simulink model "IndustrialMicrogrid"  (R2025a)
settings: Solver=FixedStepAuto  StartTime=0.0  StopTime=8  FixedStep=Ts  RelTol=1e-3
PostLoadFcn:
  | IndustrialMicrogridInputData
  | GfmGridFormingConverterInputParameters
model workspace (MAT data in the model file):
  caseNum = 2
undefined symbols (not defined in the file): base, BESS, DiscIntNeverNeededParam, grid, Grid, gridInverter, machine, microgrid, PV, PVInverter, PVTransformer, scrFactorRg, scrFactorXg, transformer, Transition_and_Dispatch_ControlModeType, Ts
libraries: ee_lib x126, fl_lib x91, eeGeneralControl x73, nesl_utility x50, nesl_utility_internal x46, simulink x30, eeTransforms x11, eeSinusoidalMeasurementV2 x5, eeTotalHarmonicDistorsion x4, slpidlib x3, simulink_extras x2, eePowerMeasurement x2
(part 3 of 12)

== system IndustrialMicrogrid/MG1 Drilling Loads/Subsystem2 ==
  ASM measurement : ee_lib/Electromechanical/Asynchronous/Induction Machine Measurement  output_idx=11
      settings: InternalSimscapePortConfiguration="{\"Bottom\":[],\"Left\":[{\"id\":\"pu_input\",\"label\":\"pu\",\"type\":\"input\"}],\"Right\":[{\"id\":\"pu_output\",\"label\":\"o\",\"type\":\"output\"}],\"Top\":[]}"
  ASM measurement1 : ee_lib/Electromechanical/Asynchronous/Induction Machine Measurement  output_idx=12
      settings: InternalSimscapePortConfiguration="{\"Bottom\":[],\"Left\":[{\"id\":\"pu_input\",\"label\":\"pu\",\"type\":\"input\"}],\"Right\":[{\"id\":\"pu_output\",\"label\":\"o\",\"type\":\"output\"}],\"Top\":[]}"
  ASM measurement2 : ee_lib/Electromechanical/Asynchronous/Induction Machine Measurement  output_idx=12
      settings: InternalSimscapePortConfiguration="{\"Bottom\":[],\"Left\":[{\"id\":\"pu_input\",\"label\":\"pu\",\"type\":\"input\"}],\"Right\":[{\"id\":\"pu_output\",\"label\":\"o\",\"type\":\"output\"}],\"Top\":[]}"
  Asynchronous Machine Squirrel Cage (fundamental) : ee_lib/Electromechanical/Asynchronous/Induction Machine Squirrel Cage  port_option=ee.enum.threePhasePort.composite  SRated=132000 V*A  VRated=microgrid.unitSubstationVoltage V  FRated=grid.frequency Hz  nPolePairs=2  param_unit=ee.enum.unit.si  squirrel_cage=ee.enum.squirrelcage.Single  zero_sequence=ee.enum.park.zerosequence.exclude  initialization_option=ee.enum.asm.initialization.fluxvariables  Rs=0.016744 Ohm  Xls=0.035490 Ohm  pu_Rs=0.0258  pu_Lls=0.0413  Rrd=0.009857 Ohm  Xlrd=0.04280 Ohm  pu_Rrd=0.0145  pu_Llrd=0.0424  Rrd1=0.28 Ohm  Xlrd1=0.82 Ohm  Rrd2=0.28 Ohm  Xlrd2=0.82 Ohm  pu_Rrd1=0.0290  pu_Llrd1=0.0848  pu_Rrd2=0.0290  pu_Llrd2=0.0848  Xm=111.90 Ohm  pu_Lm=1.7562  X0=0.4 Ohm  pu_L0=0.0413  saturation_option=ee.enum.saturation.exclude  saturation_i=[0, 4, 9, 18, 25, 34, 50, 68, 95, 120] A  saturation_v=[0, 88, 154, 198, 220, 242, 264, 286, 308, 327] V  pu_saturation_i=[0, .176, .396, .792, 1.1, 1.496, 2.2, 2.992, 4.18, 5.28]  pu_saturation_v=[0, .4, .7, .9, 1, 1.1, 1.2, 1.3, 1.4, 1.4864]  connection_option=ee.enum.Connection.delta1  angular_position_specify=off  angular_position_priority=None  angular_position=0 deg  angular_position_nominal_specify=off  angular_position_nominal_value=1  angular_position_nominal_unit=deg  pu_psids_specify=off  pu_psids_priority=None  pu_psids=0  pu_psids_nominal_specify=off  pu_psids_nominal_value=1  pu_psids_nominal_unit=1  pu_psiqs_specify=off  pu_psiqs_priority=None  pu_psiqs=0  pu_psiqs_nominal_specify=off  pu_psiqs_nominal_value=1  pu_psiqs_nominal_unit=1  pu_psi0s_specify=off  pu_psi0s_priority=None  pu_psi0s=0  pu_psi0s_nominal_specify=off  pu_psi0s_nominal_value=1  pu_psi0s_nominal_unit=1  pu_psidr_specify=off  pu_psidr_priority=None  pu_psidr=0  pu_psidr_nominal_specify=off  pu_psidr_nominal_value=1  pu_psidr_nominal_unit=1  pu_psiqr_specify=off  pu_psiqr_priority=None  pu_psiqr=0  pu_psiqr_nominal_specify=off  pu_psiqr_nominal_value=1  pu_psiqr_nominal_unit=1  pu_psidr1_specify=off  pu_psidr1_priority=None  pu_psidr1=0  pu_psidr1_nominal_specify=off  pu_psidr1_nominal_value=1  pu_psidr1_nominal_unit=1  pu_psiqr1_specify=off  pu_psiqr1_priority=None  pu_psiqr1=0  pu_psiqr1_nominal_specify=off  pu_psiqr1_nominal_value=1  pu_psiqr1_nominal_unit=1  pu_psidr2_specify=off  pu_psidr2_priority=None  pu_psidr2=0  pu_psidr2_nominal_specify=off  pu_psidr2_nominal_value=1  pu_psidr2_nominal_unit=1  pu_psiqr2_specify=off  pu_psiqr2_priority=None  pu_psiqr2=0  pu_psiqr2_nominal_specify=off  pu_psiqr2_nominal_value=1  pu_psiqr2_nominal_unit=1  psids_specify=off  psids_priority=None  psids=0 Wb  psids_nominal_specify=off  psids_nominal_value=1  psids_nominal_unit=Wb  psiqs_specify=off  psiqs_priority=None  psiqs=0 Wb  psiqs_nominal_specify=off  psiqs_nominal_value=1  psiqs_nominal_unit=Wb  psi0s_specify=off  psi0s_priority=None  psi0s=0 Wb  psi0s_nominal_specify=off  psi0s_nominal_value=1  psi0s_nominal_unit=Wb  psidr_specify=off  psidr_priority=None  psidr=0 Wb  psidr_nominal_specify=off  psidr_nominal_value=1  psidr_nominal_unit=Wb  psiqr_specify=off  psiqr_priority=None  psiqr=0 Wb  psiqr_nominal_specify=off  psiqr_nominal_value=1  psiqr_nominal_unit=Wb  psidr1_specify=off  psidr1_priority=None  psidr1=0 Wb  psidr1_nominal_specify=off  psidr1_nominal_value=1  psidr1_nominal_unit=Wb  psiqr1_specify=off  psiqr1_priority=None  psiqr1=0 Wb  psiqr1_nominal_specify=off  psiqr1_nominal_value=1  psiqr1_nominal_unit=Wb  psidr2_specify=off  psidr2_priority=None  psidr2=0 Wb  psidr2_nominal_specify=off  psidr2_nominal_value=1  psidr2_nominal_unit=Wb  psiqr2_specify=off  psiqr2_priority=None  psiqr2=0 Wb  psiqr2_nominal_specify=off  psiqr2_nominal_value=1  psiqr2_nominal_unit=Wb  slip_specify=off  slip_priority=None  slip=0  slip_nominal_specify=off  slip_nominal_value=1  slip_nominal_unit=1  real_power_generated_specify=off  real_power_generated_priority=None  real_power_generated=0 W  real_power_generated_nominal_specify=off  real_power_generated_nominal_value=1  real_power_generated_nominal_unit=W  mechanical_power_consumed_specify=off  mechanical_power_consumed_priority=None  mechanical_power_consumed=0 W  mechanical_power_consumed_nominal_specify=off  mechanical_power_consumed_nominal_value=1  mechanical_power_consumed_nominal_unit=W  Tmeas=298.15 K  alpha=3.93e-3 1/K  alpha_cage=4.4e-3 1/K  stator_thermal_mass=100 J/K  rotor_thermal_mass=200 J/K  temperatureA_specify=off  temperatureA_priority=High  temperatureA=25 degC  temperatureA_nominal_specify=off  temperatureA_nominal_value=1  temperatureA_nominal_unit=degC  temperatureB_specify=off  temperatureB_priority=High  temperatureB=25 degC  temperatureB_nominal_specify=off  temperatureB_nominal_value=1  temperatureB_nominal_unit=degC  temperatureC_specify=off  temperatureC_priority=High  temperatureC=25 degC  temperatureC_nominal_specify=off  temperatureC_nominal_value=1  temperatureC_nominal_unit=degC  temperatureR_specify=off  temperatureR_priority=High  temperatureR=25 degC  temperatureR_nominal_specify=off  temperatureR_nominal_value=1  temperatureR_nominal_unit=degC
      settings: InternalSimscapePortConfiguration="{\"Bottom\":[],\"Left\":[{\"id\":\"R\",\"label\":\"R\",\"type\":\"foundation.mechanical.rotational.rotational\"},{\"id\":\"C\",\"label\":\"C\",\"type\":\"foundation.mechanical.rotational.rotational\"}],\"Right\":[{\"id\":\"pu_output\",\"label\":\"pu\",\"type\":\"output\"},{\"id\":\"N1\",\"label\":\"~1\",\"type\":\"foundation.electrical.three_phase\"},{\"id\":\"N2\",\"label\":\"~2\",\"type\":\"foundation.electrical.three_phase\"}],\"Top\":[]}"
  Electrical Reference1 : fl_lib/Electrical/Electrical Elements/Electrical Reference
  Generator : Scope  NumInputPorts=3
      settings: TimeSpan=60  ActiveDisplayYMinimum=-4.80755  ActiveDisplayYMaximum=1.91952  DataLoggingVariableName=ScopeData2  DataLoggingSaveFormat=Array
  Generator Sign Convention : Gain  Gain=-1
  Generator Sign Convention1 : Gain  Gain=-1
  Neutral Port (Three-Phase) : ee_lib/Connectors & References/Neutral Port (Three-Phase)  G_parasitic=1e-12 1/Ohm
      settings: InternalSimscapePortConfiguration="{\"Bottom\":[],\"Left\":[{\"id\":\"N\",\"label\":\"~\",\"type\":\"foundation.electrical.three_phase\"}],\"Right\":[{\"id\":\"n\",\"label\":\"n\",\"type\":\"foundation.electrical.electrical\"}],\"Top\":[]}"
  PS-Simulink Converter1 : nesl_utility/PS-Simulink Converter  PhysicalDomain=network_engine_domain  SubClassName=ps_output  LeftPortType=input  RightPortType=output  PseudoPeriodic=off  Frequencies=[]  VectorFormat=1-D array  Unit=1  AffineConversion=off
  PS-Simulink Converter2 : nesl_utility/PS-Simulink Converter  PhysicalDomain=network_engine_domain  SubClassName=ps_output  LeftPortType=input  RightPortType=output  PseudoPeriodic=off  Frequencies=[]  VectorFormat=1-D array  Unit=1  AffineConversion=off
  PS-Simulink Converter3 : nesl_utility/PS-Simulink Converter  PhysicalDomain=network_engine_domain  SubClassName=ps_output  LeftPortType=input  RightPortType=output  PseudoPeriodic=off  Frequencies=[]  VectorFormat=1-D array  Unit=1  AffineConversion=off
  Subsystem : Subsystem
  Conn2 : PMIOPort  Side=Right
  wires:
  PS-Simulink Converter3/1 -> Generator/3
  Generator Sign Convention1/1 -> Generator/2  "Reactive Power, pu"
  PS-Simulink Converter2/1 -> Generator Sign Convention/1
  Generator Sign Convention/1 -> Generator/1  "Real Power, pu"
  PS-Simulink Converter1/1 -> Generator Sign Convention1/1
  connections:
  ASM measurement1/RConn1 -- PS-Simulink Converter1/LConn1
  PS-Simulink Converter3/LConn1 -- ASM measurement2/RConn1
  Asynchronous Machine Squirrel Cage (fundamental)/RConn3 -- Neutral Port (Three-Phase)/LConn1
  Asynchronous Machine Squirrel Cage (fundamental)/RConn2 -- Conn2/RConn1
  ASM measurement/RConn1 -- PS-Simulink Converter2/LConn1
  Neutral Port (Three-Phase)/RConn1 -- Electrical Reference1/LConn1
  Subsystem/LConn1 -- Asynchronous Machine Squirrel Cage (fundamental)/LConn1
  Subsystem/LConn2 -- Asynchronous Machine Squirrel Cage (fundamental)/LConn2
  ASM measurement1/LConn1 -- ASM measurement2/LConn1 -- Asynchronous Machine Squirrel Cage (fundamental)/RConn1 -- ASM measurement/LConn1

== system IndustrialMicrogrid/MG1 Portable Substation/Circuit Breaker1 ==
  BRK : Inport
  Data Type Conversion : DataTypeConversion  OutDataTypeStr=double  SaturateOnIntegerOverflow=off  RndMeth=Floor
  Open Resistance : Gain  Gain=1e5
  Phase Splitter : ee_lib/Connectors & References/Phase Splitter
  Phase Splitter1 : ee_lib/Connectors & References/Phase Splitter
  Simulink-PS Converter : nesl_utility/Simulink-PS Converter  PhysicalDomain=network_engine_domain  SubClassName=ps_input  LeftPortType=input  RightPortType=output  PseudoPeriodic=off  Frequencies=[]  NoiseDistribution=none  NoiseParameters=[]  Unit=1  AffineConversion=off  FilteringAndDerivatives=provide  SimscapeFilterOrder=1  InputFilterTimeConstant=0.001  UdotUserProvided=0
  Variable Resistor : fl_lib/Electrical/Electrical Elements/Variable Resistor  Rmin=1e-3 Ohm  thermalEnable=false  thermal_mass=1 J/K  i_specify=off  i_priority=None  i=0 A  i_nominal_specify=off  i_nominal_value=1  i_nominal_unit=A  v_specify=off  v_priority=None  v=0 V  v_nominal_specify=off  v_nominal_value=1  v_nominal_unit=V  T_specify=off  T_priority=None  T=300 K  T_nominal_specify=off  T_nominal_value=1  T_nominal_unit=K
  Variable Resistor1 : fl_lib/Electrical/Electrical Elements/Variable Resistor  Rmin=1e-3 Ohm  thermalEnable=false  thermal_mass=1 J/K  i_specify=off  i_priority=None  i=0 A  i_nominal_specify=off  i_nominal_value=1  i_nominal_unit=A  v_specify=off  v_priority=None  v=0 V  v_nominal_specify=off  v_nominal_value=1  v_nominal_unit=V  T_specify=off  T_priority=None  T=300 K  T_nominal_specify=off  T_nominal_value=1  T_nominal_unit=K
  Variable Resistor2 : fl_lib/Electrical/Electrical Elements/Variable Resistor  Rmin=1e-3 Ohm  thermalEnable=false  thermal_mass=1 J/K  i_specify=off  i_priority=None  i=0 A  i_nominal_specify=off  i_nominal_value=1  i_nominal_unit=A  v_specify=off  v_priority=None  v=0 V  v_nominal_specify=off  v_nominal_value=1  v_nominal_unit=V  T_specify=off  T_priority=None  T=300 K  T_nominal_specify=off  T_nominal_value=1  T_nominal_unit=K
  In : PMIOPort  Side=Left
  ~ : PMIOPort  Port=2  Side=Right
  wires:
  Data Type Conversion/1 -> Open Resistance/1
  BRK/1 -> Data Type Conversion/1
  Open Resistance/1 -> Simulink-PS Converter/1
  connections:
  Phase Splitter1/RConn2 -- Variable Resistor1/RConn1
  Variable Resistor1/LConn2 -- Phase Splitter/RConn2
  Phase Splitter1/RConn3 -- Variable Resistor2/RConn1
  Phase Splitter/RConn1 -- Variable Resistor/LConn2
  Variable Resistor2/LConn2 -- Phase Splitter/RConn3
  Phase Splitter1/RConn1 -- Variable Resistor/RConn1
  Phase Splitter1/LConn1 -- ~/RConn1
  Variable Resistor/LConn1 -- Simulink-PS Converter/RConn1 -- Variable Resistor2/LConn1 -- Variable Resistor1/LConn1
  Phase Splitter/LConn1 -- In/RConn1

== system IndustrialMicrogrid/MG1 Primary Substation/BESS and Controller ==
  CntrlRmIN : Inport
  Vref : Inport  Port=2
  f0 : Inport  Port=3
  PQref : Inport  Port=4
  BESS : Subsystem
      settings: PortSchema="{\"entries\":[{\"content\":{\"sides\":[{\"content\":{\"connectorIds\":[\"LConn1\"]},\"type\":\"ConnectorPlacement.EquallySpacedRectSide\",\"uuid\":\"2696dcad-9c9f-4771-9a46-e4805fbfd4e9\"},{\"content\":{\"connectorIds\":[\"In1\",\"In2\",\"In3\",\"In4\"],\"side\":\"RIGHT\"},\"type\":\"ConnectorPlacement.EquallySpacedRectSide\",\"uuid\":\"645d6df5-6573-4261-af42-019db177e35c\"},{\"content\":{\"side\":\"TOP\"},\"type\":\"ConnectorPlacement.EquallySpacedRectSide\",\"uuid\":\"6dbeb1fb-6f20-4035-89b5-3497a08373ed\"}]},\"type\":\"ConnectorPlacement.EquallySpacedConnector\",\"uuid\":\"8e6ce7c3-5a23-40aa-ad05-ea5cef07dce4\"}],\"packageUris\":[\"http://schema.mathworks.com/mf0/Connector/R2020b\"],\"version\":\"1.0\"}"
  "BESS Converter Measurement " : Subsystem
  BESS output filter and transformer1 : Subsystem
  Gain : Gain  Gain=1/grid.frequency
  ~ : PMIOPort  Side=Left
  mBESS : Outport
  wires:
  PQref/1 -> BESS/2(PQref)
  "BESS Converter Measurement "/1(mBESS1) -> mBESS/1
  Vref/1 -> BESS/3(Vref)
  f0/1 -> Gain/1
  CntrlRmIN/1 -> BESS/1(CntrlRmIN1)
  Gain/1 -> BESS/4(f0)
  connections:
  BESS output filter and transformer1/RConn1 -- "BESS Converter Measurement "/LConn1
  BESS/LConn1 -- BESS output filter and transformer1/LConn1
  ~/RConn1 -- "BESS Converter Measurement "/RConn1

== system IndustrialMicrogrid/MG1 Primary Substation/Circuit Breaker1 ==
  BRK : Inport
  Data Type Conversion : DataTypeConversion  OutDataTypeStr=double  SaturateOnIntegerOverflow=off  RndMeth=Floor
  Open Resistance : Gain  Gain=1e5
  Phase Splitter : ee_lib/Connectors & References/Phase Splitter
  Phase Splitter1 : ee_lib/Connectors & References/Phase Splitter
  Simulink-PS Converter : nesl_utility/Simulink-PS Converter  PhysicalDomain=network_engine_domain  SubClassName=ps_input  LeftPortType=input  RightPortType=output  PseudoPeriodic=off  Frequencies=[]  NoiseDistribution=none  NoiseParameters=[]  Unit=1  AffineConversion=off  FilteringAndDerivatives=provide  SimscapeFilterOrder=1  InputFilterTimeConstant=0.001  UdotUserProvided=0
  Variable Resistor : fl_lib/Electrical/Electrical Elements/Variable Resistor  Rmin=1e-3 Ohm  thermalEnable=false  thermal_mass=1 J/K  i_specify=off  i_priority=None  i=0 A  i_nominal_specify=off  i_nominal_value=1  i_nominal_unit=A  v_specify=off  v_priority=None  v=0 V  v_nominal_specify=off  v_nominal_value=1  v_nominal_unit=V  T_specify=off  T_priority=None  T=300 K  T_nominal_specify=off  T_nominal_value=1  T_nominal_unit=K
  Variable Resistor1 : fl_lib/Electrical/Electrical Elements/Variable Resistor  Rmin=1e-3 Ohm  thermalEnable=false  thermal_mass=1 J/K  i_specify=off  i_priority=None  i=0 A  i_nominal_specify=off  i_nominal_value=1  i_nominal_unit=A  v_specify=off  v_priority=None  v=0 V  v_nominal_specify=off  v_nominal_value=1  v_nominal_unit=V  T_specify=off  T_priority=None  T=300 K  T_nominal_specify=off  T_nominal_value=1  T_nominal_unit=K
  Variable Resistor2 : fl_lib/Electrical/Electrical Elements/Variable Resistor  Rmin=1e-3 Ohm  thermalEnable=false  thermal_mass=1 J/K  i_specify=off  i_priority=None  i=0 A  i_nominal_specify=off  i_nominal_value=1  i_nominal_unit=A  v_specify=off  v_priority=None  v=0 V  v_nominal_specify=off  v_nominal_value=1  v_nominal_unit=V  T_specify=off  T_priority=None  T=300 K  T_nominal_specify=off  T_nominal_value=1  T_nominal_unit=K
  In : PMIOPort  Side=Left
  ~ : PMIOPort  Port=2  Side=Right
  wires:
  Data Type Conversion/1 -> Open Resistance/1
  Open Resistance/1 -> Simulink-PS Converter/1
  BRK/1 -> Data Type Conversion/1
  connections:
  Phase Splitter1/RConn2 -- Variable Resistor1/RConn1
  Variable Resistor1/LConn2 -- Phase Splitter/RConn2
  Phase Splitter1/RConn3 -- Variable Resistor2/RConn1
  Phase Splitter/RConn1 -- Variable Resistor/LConn2
  Variable Resistor2/LConn2 -- Phase Splitter/RConn3
  Phase Splitter1/RConn1 -- Variable Resistor/RConn1
  Phase Splitter1/LConn1 -- ~/RConn1
  Variable Resistor/LConn1 -- Simulink-PS Converter/RConn1 -- Variable Resistor2/LConn1 -- Variable Resistor1/LConn1
  Phase Splitter/LConn1 -- In/RConn1

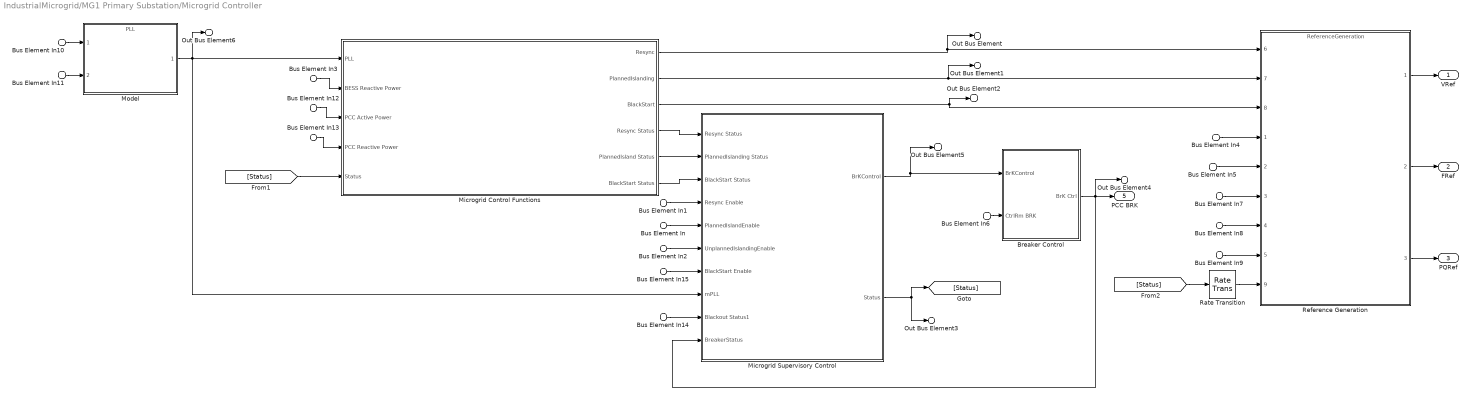
== system IndustrialMicrogrid/MG1 Primary Substation/Microgrid Controller ==
  Bus Element In3 : Inport  PortName=CtrlRm  Element=BESSReactivePower
  Bus Element In9 : Inport  PortName=CtrlRm  Element=PowerCmd
  Bus Element In : Inport  PortName=CtrlRm  Element=plannedIslanding
  Bus Element In2 : Inport  PortName=CtrlRm  Element=unplannedIslanding
  Bus Element In6 : Inport  PortName=CtrlRm  Element=BRKcontrol
  Bus Element In1 : Inport  PortName=CtrlRm  Element=Resync
  Bus Element In4 : Inport  PortName=CtrlRm  Element=BESS.PRef
  Bus Element In5 : Inport  PortName=CtrlRm  Element=BESS.QRef
  Bus Element In7 : Inport  PortName=CtrlRm  Element=BESS.VRef
  Bus Element In8 : Inport  PortName=CtrlRm  Element=BESS.FRef
  Bus Element In15 : Inport  PortName=CtrlRm  Element=blackStart
  Bus Element In14 : Inport  PortName=CtrlRm  Element=blackout
  Bus Element In10 : Inport  Port=2  PortName=mPCC  Element=Grid.voltage
  Bus Element In11 : Inport  Port=2  PortName=mPCC  Element=PCC.voltage
  Bus Element In12 : Inport  Port=2  PortName=mPCC  Element=PCC.activePower
  Bus Element In13 : Inport  Port=2  PortName=mPCC  Element=PCC.reactivePower
  Breaker Control : Subsystem  mask(Breaker Control){}
      mask help: Control breaker at PCC
  Microgrid Control Functions : Subsystem
  Microgrid Supervisory Control : Subsystem
  Model : ModelReference  ModelNameDialog=PLL.slx  UsingDefaultArgumentValue=0,0,0  SimulationMode=Normal  ModelReferenceVersion=5.0  GridFrequency=gridFrequency  KiPLLController=kpPLL  KpPLLController=kiPLL
  Rate Transition : RateTransition  OutPortSampleTime=1e-3
  Reference Generation : ModelReference  ModelNameDialog=ReferenceGeneration.slx  UsingDefaultArgumentValue=0,0,0,0,0  SimulationMode=Normal  ModelReferenceVersion=5.0  GridFrequency=gridFrequency  pUpperLimit=pUpperLimit  pLowerLimit=pLowerLimit  qUpperLimit=qUpperLimit  qLowerLimit=qLowerLimit
      settings: PortSchema="{\"entries\":[{\"content\":{\"sides\":[{\"content\":{\"connectorIds\":[\"In6\",\"In7\",\"In8\",\"In1\",\"In2\",\"In3\",\"In4\",\"In5\",\"In9\"]},\"type\":\"ConnectorPlacement.EquallySpacedRectSide\",\"uuid\":\"e872b833-49f6-4912-b4b3-51343786db27\"},{\"content\":{\"connectorIds\":[\"Out1\",\"Out2\",\"Out3\"],\"side\":\"RIGHT\"},\"type\":\"ConnectorPlacement.EquallySpacedRectSide\",\"uuid\":\"d01ecec0-b655-4b5d-a34d-324f522879ad\"},{\"content\":{\"side\":\"TOP\"},\"type\":\"ConnectorPlacement.EquallySpacedRectSide\",\"uuid\":\"07b88f4e-1122-4691-94e1-fc20c2cbb47d\"}]},\"type\":\"ConnectorPlacement.EquallySpacedConnector\",\"uuid\":\"8d1da379-bdae-48c1-83d9-0dc3b93882b1\"}],\"packageUris\":[\"http://schema.mathworks.com/mf0/Connector/R2020b\"],\"version\":\"1.0\"}"
  VRef : Outport
  FRef : Outport  Port=2
  PQRef : Outport  Port=3
  Out Bus Element : Outport  Port=4  PortName=MGController  Element=Resync
  Out Bus Element1 : Outport  Port=4  PortName=MGController  Element=PlannedIslanding
  Out Bus Element2 : Outport  Port=4  PortName=MGController  Element=BlackStart
  Out Bus Element3 : Outport  Port=4  PortName=MGController  Element=Status
  Out Bus Element4 : Outport  Port=4  PortName=MGController  Element=BRK Status
  Out Bus Element6 : Outport  Port=4  PortName=MGController  Element=mPLL
  Out Bus Element5 : Outport  Port=4  PortName=MGController  Element=BrKControl
  PCC BRK : Outport  Port=5
  wires:
  Bus Element In7/1 -> Reference Generation/3
  Reference Generation/2 -> FRef/1
  Bus Element In8/1 -> Reference Generation/4
  Bus Element In3/1 -> Microgrid Control Functions/2(BESS Reactive Power)
  Reference Generation/1 -> VRef/1
  Reference Generation/3 -> PQRef/1
  Bus Element In12/1 -> Microgrid Control Functions/3(PCC Active Power)
  Bus Element In4/1 -> Reference Generation/1
  Bus Element In13/1 -> Microgrid Control Functions/4(PCC Reactive Power)
  Bus Element In10/1 -> Model/1
  Bus Element In5/1 -> Reference Generation/2
  Bus Element In2/1 -> Microgrid Supervisory Control/6(UnplannedIslandingEnable)
  Bus Element In/1 -> Microgrid Supervisory Control/5(PlannedIslandEnable)
  Bus Element In11/1 -> Model/2
  Bus Element In9/1 -> Reference Generation/5
  Bus Element In1/1 -> Microgrid Supervisory Control/4(Resync Enable)
  Microgrid Supervisory Control/1(BrKControl) -> Out Bus Element5/1, Breaker Control/1(BrKControl)
  Bus Element In6/1 -> Breaker Control/2(CtrlRm BRK)
  Model/1 -> Out Bus Element6/1, Microgrid Control Functions/1(PLL), Microgrid Supervisory Control/8(mPLL)
  Microgrid Control Functions/2(PlannedIslanding) -> Out Bus Element1/1, Reference Generation/7
  Microgrid Control Functions/1(Resync) -> Out Bus Element/1, Reference Generation/6
  Breaker Control/1(BrK Ctrl) -> Microgrid Supervisory Control/10(BreakerStatus), PCC BRK/1, Out Bus Element4/1
  Microgrid Control Functions/3(BlackStart) -> Out Bus Element2/1, Reference Generation/8
  Microgrid Supervisory Control/2(Status) -> Out Bus Element3/1, [Status]
  [Status] -> Microgrid Control Functions/5(Status)
  [Status] -> Rate Transition/1
  Rate Transition/1 -> Reference Generation/9
  Bus Element In15/1 -> Microgrid Supervisory Control/7(BlackStart Enable)
  Microgrid Control Functions/4(Resync Status) -> Microgrid Supervisory Control/1(Resync Status)
  Microgrid Control Functions/5(PlannedIsland Status) -> Microgrid Supervisory Control/2(PlannedIslanding Status)
  Microgrid Control Functions/6(BlackStart Status) -> Microgrid Supervisory Control/3(BlackStart Status)
  Bus Element In14/1 -> Microgrid Supervisory Control/9(Blackout Status1)

== system IndustrialMicrogrid/MG1 Primary Substation/PCC Measurements and PCC Breaker ==
  cBreaker : Inport
  Bus Creator : BusCreator  Inputs=2
  Circuit Breaker : Subsystem
  Grid Current Measurement : Subsystem
  Grid Power Measurement : Subsystem
  ~ : PMIOPort  Side=Left
  "~ " : PMIOPort  Port=2  Side=Right
  " mPCC" : Outport
  wires:
  Grid Power Measurement/1(PCC) -> Bus Creator/2  "PCC"
  Bus Creator/1 -> " mPCC"/1
  cBreaker/1 -> Circuit Breaker/1(BRK)
  Grid Current Measurement/1(Grid) -> Bus Creator/1  "Grid"
  connections:
  ~/RConn1 -- Grid Current Measurement/LConn1
  Circuit Breaker/RConn1 -- Grid Power Measurement/LConn1
  Grid Power Measurement/RConn1 -- "~ "/RConn1
  Circuit Breaker/LConn1 -- Grid Current Measurement/RConn1

== system IndustrialMicrogrid/MG1 Primary Substation/Transformer and Disconnectors ==
  Connectors : ee_lib/Passive/RLC Assemblies/RLC (Three-Phase)  port_option=ee.enum.threePhasePort.composite  component_structure=ee.enum.rlc.structure.R  R=grid.connectorResistance*100 Ohm  L=0.01 H  C=1e-6 F  R_parasitic=1e-6 Ohm  G_parasitic=1e-6 1/Ohm  IL_specify=on  IL_priority=High  IL=[0, 0, 0] A  IL_nominal_specify=off  IL_nominal_value=1  IL_nominal_unit=A  VC_specify=off  VC_priority=High  VC=[0, 0, 0] V  VC_nominal_specify=off  VC_nominal_value=1  VC_nominal_unit=V
      settings: InternalSimscapePortConfiguration="{\"Bottom\":[],\"Left\":[{\"id\":\"N1\",\"label\":\"~1\",\"type\":\"foundation.electrical.three_phase\"}],\"Right\":[{\"id\":\"N2\",\"label\":\"~2\",\"type\":\"foundation.electrical.three_phase\"}],\"Top\":[]}"
  Two-Winding Transformer (Three-Phase)1 : ee_lib/Passive/Transformers/Two-Winding Transformer (Three-Phase)  SRated=grid.transformerRating A*V  FRated=grid.frequency Hz  Winding1Connection=ee.enum.windingconnection.Y  VRated1=grid.transformerPrimaryVoltage V  Winding2Connection=ee.enum.windingconnection.Y  VRated2=grid.transformerSecondaryVoltage V  CoreType=ee.enum.coretype.threelimb  pu_Rw1=grid.primaryResistance  pu_Rw2=grid.primaryReactance  leakage_reactance_option=ee.enum.transformer_leakage.include  pu_Xl1=grid.secondaryResistance  pu_Xl2=grid.secondaryReactance  magnetizing_resistance_option=ee.enum.transformer_magnetizingResistance.include  pu_Rm=500  magnetizing_reactance_option=ee.enum.transformer_magnetizingReactance.include  saturation_option=ee.enum.transformer_saturation.exclude  pu_Xm=500  current_data=[0, .002, 1, 2]  magnetic_flux_data=[0, 1.2, 1.5, 1.51]  pu_X0=0.5  i1_specify=on  i1_priority=None  i1=[0, 0, 0] A  i1_nominal_specify=off  i1_nominal_value=1  i1_nominal_unit=A  i2_specify=on  i2_priority=None  i2=[0, 0, 0] A  i2_nominal_specify=off  i2_nominal_value=1  i2_nominal_unit=A  phi_specify=off  phi_priority=None  phi=[0, 0, 0]  phi_nominal_specify=off  phi_nominal_value=1  phi_nominal_unit=1  power_dissipated_specify=off  power_dissipated_priority=None  power_dissipated=0 W  power_dissipated_nominal_specify=off  power_dissipated_nominal_value=1  power_dissipated_nominal_unit=W
      settings: InternalSimscapePortConfiguration="{\"Bottom\":[],\"Left\":[{\"id\":\"N1\",\"label\":\"~1\",\"type\":\"foundation.electrical.three_phase\"}],\"Right\":[{\"id\":\"N2\",\"label\":\"~2\",\"type\":\"foundation.electrical.three_phase\"}],\"Top\":[]}"
  "~ " : PMIOPort  Side=Right
  ~ : PMIOPort  Port=2  Side=Left
  connections:
  ~/RConn1 -- Two-Winding Transformer (Three-Phase)1/LConn1
  Connectors/RConn1 -- "~ "/RConn1
  Connectors/LConn1 -- Two-Winding Transformer (Three-Phase)1/RConn1

== system IndustrialMicrogrid/MG1 Unit Substation/Circuit Breaker1 ==
  BRK : Inport
  Data Type Conversion : DataTypeConversion  OutDataTypeStr=double  SaturateOnIntegerOverflow=off  RndMeth=Floor
  Open Resistance : Gain  Gain=1e5
  Phase Splitter : ee_lib/Connectors & References/Phase Splitter
  Phase Splitter1 : ee_lib/Connectors & References/Phase Splitter
  Simulink-PS Converter : nesl_utility/Simulink-PS Converter  PhysicalDomain=network_engine_domain  SubClassName=ps_input  LeftPortType=input  RightPortType=output  PseudoPeriodic=off  Frequencies=[]  NoiseDistribution=none  NoiseParameters=[]  Unit=1  AffineConversion=off  FilteringAndDerivatives=provide  SimscapeFilterOrder=1  InputFilterTimeConstant=0.001  UdotUserProvided=0
  Variable Resistor : fl_lib/Electrical/Electrical Elements/Variable Resistor  Rmin=1e-3 Ohm  thermalEnable=false  thermal_mass=1 J/K  i_specify=off  i_priority=None  i=0 A  i_nominal_specify=off  i_nominal_value=1  i_nominal_unit=A  v_specify=off  v_priority=None  v=0 V  v_nominal_specify=off  v_nominal_value=1  v_nominal_unit=V  T_specify=off  T_priority=None  T=300 K  T_nominal_specify=off  T_nominal_value=1  T_nominal_unit=K
  Variable Resistor1 : fl_lib/Electrical/Electrical Elements/Variable Resistor  Rmin=1e-3 Ohm  thermalEnable=false  thermal_mass=1 J/K  i_specify=off  i_priority=None  i=0 A  i_nominal_specify=off  i_nominal_value=1  i_nominal_unit=A  v_specify=off  v_priority=None  v=0 V  v_nominal_specify=off  v_nominal_value=1  v_nominal_unit=V  T_specify=off  T_priority=None  T=300 K  T_nominal_specify=off  T_nominal_value=1  T_nominal_unit=K
  Variable Resistor2 : fl_lib/Electrical/Electrical Elements/Variable Resistor  Rmin=1e-3 Ohm  thermalEnable=false  thermal_mass=1 J/K  i_specify=off  i_priority=None  i=0 A  i_nominal_specify=off  i_nominal_value=1  i_nominal_unit=A  v_specify=off  v_priority=None  v=0 V  v_nominal_specify=off  v_nominal_value=1  v_nominal_unit=V  T_specify=off  T_priority=None  T=300 K  T_nominal_specify=off  T_nominal_value=1  T_nominal_unit=K
  In : PMIOPort  Side=Left
  ~ : PMIOPort  Port=2  Side=Right
  wires:
  Data Type Conversion/1 -> Open Resistance/1
  BRK/1 -> Data Type Conversion/1
  Open Resistance/1 -> Simulink-PS Converter/1
  connections:
  Phase Splitter1/RConn2 -- Variable Resistor1/RConn1
  Variable Resistor1/LConn2 -- Phase Splitter/RConn2
  Phase Splitter1/RConn3 -- Variable Resistor2/RConn1
  Phase Splitter/RConn1 -- Variable Resistor/LConn2
  Variable Resistor2/LConn2 -- Phase Splitter/RConn3
  Phase Splitter1/RConn1 -- Variable Resistor/RConn1
  Phase Splitter1/LConn1 -- ~/RConn1
  Variable Resistor/LConn1 -- Simulink-PS Converter/RConn1 -- Variable Resistor2/LConn1 -- Variable Resistor1/LConn1
  Phase Splitter/LConn1 -- In/RConn1

== system IndustrialMicrogrid/MG1 Unit Substation/Circuit Breaker3 ==
  BRK : Inport
  Data Type Conversion : DataTypeConversion  OutDataTypeStr=double  SaturateOnIntegerOverflow=off  RndMeth=Floor
  Open Resistance : Gain  Gain=1e5
  Phase Splitter : ee_lib/Connectors & References/Phase Splitter
  Phase Splitter1 : ee_lib/Connectors & References/Phase Splitter
  Simulink-PS Converter : nesl_utility/Simulink-PS Converter  PhysicalDomain=network_engine_domain  SubClassName=ps_input  LeftPortType=input  RightPortType=output  PseudoPeriodic=off  Frequencies=[]  NoiseDistribution=none  NoiseParameters=[]  Unit=1  AffineConversion=off  FilteringAndDerivatives=provide  SimscapeFilterOrder=1  InputFilterTimeConstant=0.001  UdotUserProvided=0
  Variable Resistor : fl_lib/Electrical/Electrical Elements/Variable Resistor  Rmin=1e-3 Ohm  thermalEnable=false  thermal_mass=1 J/K  i_specify=off  i_priority=None  i=0 A  i_nominal_specify=off  i_nominal_value=1  i_nominal_unit=A  v_specify=off  v_priority=None  v=0 V  v_nominal_specify=off  v_nominal_value=1  v_nominal_unit=V  T_specify=off  T_priority=None  T=300 K  T_nominal_specify=off  T_nominal_value=1  T_nominal_unit=K
  Variable Resistor1 : fl_lib/Electrical/Electrical Elements/Variable Resistor  Rmin=1e-3 Ohm  thermalEnable=false  thermal_mass=1 J/K  i_specify=off  i_priority=None  i=0 A  i_nominal_specify=off  i_nominal_value=1  i_nominal_unit=A  v_specify=off  v_priority=None  v=0 V  v_nominal_specify=off  v_nominal_value=1  v_nominal_unit=V  T_specify=off  T_priority=None  T=300 K  T_nominal_specify=off  T_nominal_value=1  T_nominal_unit=K
  Variable Resistor2 : fl_lib/Electrical/Electrical Elements/Variable Resistor  Rmin=1e-3 Ohm  thermalEnable=false  thermal_mass=1 J/K  i_specify=off  i_priority=None  i=0 A  i_nominal_specify=off  i_nominal_value=1  i_nominal_unit=A  v_specify=off  v_priority=None  v=0 V  v_nominal_specify=off  v_nominal_value=1  v_nominal_unit=V  T_specify=off  T_priority=None  T=300 K  T_nominal_specify=off  T_nominal_value=1  T_nominal_unit=K
  In : PMIOPort  Side=Left
  ~ : PMIOPort  Port=2  Side=Right
  wires:
  Data Type Conversion/1 -> Open Resistance/1
  BRK/1 -> Data Type Conversion/1
  Open Resistance/1 -> Simulink-PS Converter/1
  connections:
  Phase Splitter1/RConn2 -- Variable Resistor1/RConn1
  Variable Resistor1/LConn2 -- Phase Splitter/RConn2
  Phase Splitter1/RConn3 -- Variable Resistor2/RConn1
  Phase Splitter/RConn1 -- Variable Resistor/LConn2
  Variable Resistor2/LConn2 -- Phase Splitter/RConn3
  Phase Splitter1/RConn1 -- Variable Resistor/RConn1
  Phase Splitter1/LConn1 -- ~/RConn1
  Variable Resistor/LConn1 -- Simulink-PS Converter/RConn1 -- Variable Resistor2/LConn1 -- Variable Resistor1/LConn1
  Phase Splitter/LConn1 -- In/RConn1

== system IndustrialMicrogrid/MG2 PV Plant/(500KWp PV) ==
  In Bus Element3 : Inport  PortName=Vbus
  Constant : Constant  Value=0  SampleTime=Ts
  Constant1 : Constant  Value=0  SampleTime=Ts
  Constant2 : Constant  Value=1000  VectorParams1D=off  SampleTime=-1
  Current and Voltage Sensor (Three-Phase)3 : ee_lib/Sensors & Transducers/Current and Voltage Sensor (Three-Phase)  vMeasurementType=ee.enum.vmeasurement.lg  outputUnit=ee.enum.unit.pu  SRated=PV.MVABaseNew A*V  VRated=PV.kVBaseNew V  I_specify=off  I_priority=None  I=[0, 0, 0] A  I_nominal_specify=off  I_nominal_value=1  I_nominal_unit=A  V_specify=off  V_priority=None  V=[0, 0, 0] V  V_nominal_specify=off  V_nominal_value=1  V_nominal_unit=V
      settings: InternalSimscapePortConfiguration="{\"Bottom\":[],\"Left\":[{\"id\":\"N1\",\"label\":\"~1\",\"type\":\"foundation.electrical.three_phase\"}],\"Right\":[{\"id\":\"V_output\",\"label\":\"V\",\"type\":\"output\"},{\"id\":\"I_output\",\"label\":\"I\",\"type\":\"output\"},{\"id\":\"N2\",\"label\":\"~2\",\"type\":\"foundation.electrical.three_phase\"}],\"Top\":[]}"
  L Filter2 : ee_lib/Passive/RLC Assemblies/RLC (Three-Phase)  port_option=ee.enum.threePhasePort.composite  component_structure=ee.enum.rlc.structure.SeriesRL  R=0.1 Ohm  L=PVInverter.l*3 H  C=1e-6 F  R_parasitic=0 Ohm  G_parasitic=0 1/Ohm  IL_specify=on  IL_priority=None  IL=[0, 0, 0] A  IL_nominal_specify=off  IL_nominal_value=1  IL_nominal_unit=A  VC_specify=off  VC_priority=High  VC=[0, 0, 0] V  VC_nominal_specify=off  VC_nominal_value=1  VC_nominal_unit=V
      settings: InternalSimscapePortConfiguration="{\"Bottom\":[],\"Left\":[{\"id\":\"N1\",\"label\":\"~1\",\"type\":\"foundation.electrical.three_phase\"}],\"Right\":[{\"id\":\"N2\",\"label\":\"~2\",\"type\":\"foundation.electrical.three_phase\"}],\"Top\":[]}"
  Low-Pass Filter (Discrete or Continuous) : eeGeneralControl/Low-Pass Filter (Discrete or Continuous)  K=1  T=0.1  B=inf  A=-inf  init_option=Inherited from block input  x0=0  Ts=-1
  Low-Pass Filter (Discrete or Continuous)1 : eeGeneralControl/Low-Pass Filter (Discrete or Continuous)  K=1  T=0.1  B=inf  A=-inf  init_option=Inherited from block input  x0=0  Ts=-1
  Measurement2 : Subsystem
  PS-Simulink Converter : nesl_utility/PS-Simulink Converter  PhysicalDomain=network_engine_domain  SubClassName=ps_output  LeftPortType=input  RightPortType=output  PseudoPeriodic=off  Frequencies=[]  VectorFormat=inherit  Unit=MW  AffineConversion=off
  PS-Simulink Converter2 : nesl_utility/PS-Simulink Converter  PhysicalDomain=network_engine_domain  SubClassName=ps_output  LeftPortType=input  RightPortType=output  PseudoPeriodic=off  Frequencies=[]  VectorFormat=inherit  Unit=MV*A  AffineConversion=off
  PS-Simulink Converter5 : nesl_utility/PS-Simulink Converter  PhysicalDomain=network_engine_domain  SubClassName=ps_output  LeftPortType=input  RightPortType=output  PseudoPeriodic=off  Frequencies=[]  VectorFormat=inherit  Unit=inherit  AffineConversion=off
  PS-Simulink Converter6 : nesl_utility/PS-Simulink Converter  PhysicalDomain=network_engine_domain  SubClassName=ps_output  LeftPortType=input  RightPortType=output  PseudoPeriodic=off  Frequencies=[]  VectorFormat=inherit  Unit=inherit  AffineConversion=off
  PV Inverter A2 : Subsystem
  Power Sensor (Three-Phase) : ee_lib/Sensors & Transducers/Power Sensor (Three-Phase)  load_type=ee.enum.passive.type_balanced.balanced  f0=60 Hz  config=ee.enum.with_neutral.no  rho=1
      settings: InternalSimscapePortConfiguration="{\"Bottom\":[],\"Left\":[{\"id\":\"N1\",\"label\":\"~1\",\"type\":\"foundation.electrical.three_phase\"}],\"Right\":[{\"id\":\"N2\",\"label\":\"~2\",\"type\":\"foundation.electrical.three_phase\"}],\"Top\":[{\"id\":\"Pm\",\"label\":\"P\",\"type\":\"output\"},{\"id\":\"Qm\",\"label\":\"Q\",\"type\":\"output\"}]}"
  Terminator3 : Terminator
  Connection Port : PMIOPort  Side=Left
  Out Bus Element23 : Outport  PortName=PV  Element=activePower
  Out Bus Element1 : Outport  PortName=PV  Element=rectivePower
  Out Bus Element2 : Outport  PortName=PV  Element=voltage
  Out Bus Element3 : Outport  PortName=PV  Element=current
  wires:
  Constant2/1 -> PV Inverter A2/1(Insolation)
  Low-Pass Filter (Discrete or Continuous)1/1 -> Out Bus Element23/1
  Low-Pass Filter (Discrete or Continuous)/1 -> Out Bus Element1/1
  PS-Simulink Converter2/1 -> Low-Pass Filter (Discrete or Continuous)/1
  PS-Simulink Converter/1 -> Low-Pass Filter (Discrete or Continuous)1/1
  Constant/1 -> PV Inverter A2/3(LVRT)
  Measurement2/1(ipv1) -> PV Inverter A2/4(ipv1)
  PS-Simulink Converter5/1 -> Out Bus Element3/1, Measurement2/1(u)
  Constant1/1 -> PV Inverter A2/5(Q_ref)
  In Bus Element3/1 -> PV Inverter A2/2(Vbus)
  PS-Simulink Converter6/1 -> Terminator3/1, Out Bus Element2/1
  connections:
  Power Sensor (Three-Phase)/LConn3 -- PS-Simulink Converter2/LConn1
  PS-Simulink Converter/LConn1 -- Power Sensor (Three-Phase)/LConn2
  PV Inverter A2/RConn1 -- Power Sensor (Three-Phase)/LConn1
  L Filter2/LConn1 -- Power Sensor (Three-Phase)/RConn1
  L Filter2/RConn1 -- Current and Voltage Sensor (Three-Phase)3/LConn1
  PS-Simulink Converter6/LConn1 -- Current and Voltage Sensor (Three-Phase)3/RConn1
  PS-Simulink Converter5/LConn1 -- Current and Voltage Sensor (Three-Phase)3/RConn2
  Connection Port/RConn1 -- Current and Voltage Sensor (Three-Phase)3/RConn3

== system IndustrialMicrogrid/MG2 PV Plant/Circuit Breaker ==
  BRK : Inport
  Data Type Conversion : DataTypeConversion  OutDataTypeStr=double  SaturateOnIntegerOverflow=off  RndMeth=Floor
  Open Resistance : Gain  Gain=1e5
  Phase Splitter : ee_lib/Connectors & References/Phase Splitter
  Phase Splitter1 : ee_lib/Connectors & References/Phase Splitter
  Simulink-PS Converter : nesl_utility/Simulink-PS Converter  PhysicalDomain=network_engine_domain  SubClassName=ps_input  LeftPortType=input  RightPortType=output  PseudoPeriodic=off  Frequencies=[]  NoiseDistribution=none  NoiseParameters=[]  Unit=1  AffineConversion=off  FilteringAndDerivatives=provide  SimscapeFilterOrder=1  InputFilterTimeConstant=0.001  UdotUserProvided=0
  Variable Resistor : fl_lib/Electrical/Electrical Elements/Variable Resistor  Rmin=1e-3 Ohm  thermalEnable=false  thermal_mass=1 J/K  i_specify=off  i_priority=None  i=0 A  i_nominal_specify=off  i_nominal_value=1  i_nominal_unit=A  v_specify=off  v_priority=None  v=0 V  v_nominal_specify=off  v_nominal_value=1  v_nominal_unit=V  T_specify=off  T_priority=None  T=300 K  T_nominal_specify=off  T_nominal_value=1  T_nominal_unit=K
  Variable Resistor1 : fl_lib/Electrical/Electrical Elements/Variable Resistor  Rmin=1e-3 Ohm  thermalEnable=false  thermal_mass=1 J/K  i_specify=off  i_priority=None  i=0 A  i_nominal_specify=off  i_nominal_value=1  i_nominal_unit=A  v_specify=off  v_priority=None  v=0 V  v_nominal_specify=off  v_nominal_value=1  v_nominal_unit=V  T_specify=off  T_priority=None  T=300 K  T_nominal_specify=off  T_nominal_value=1  T_nominal_unit=K
  Variable Resistor2 : fl_lib/Electrical/Electrical Elements/Variable Resistor  Rmin=1e-3 Ohm  thermalEnable=false  thermal_mass=1 J/K  i_specify=off  i_priority=None  i=0 A  i_nominal_specify=off  i_nominal_value=1  i_nominal_unit=A  v_specify=off  v_priority=None  v=0 V  v_nominal_specify=off  v_nominal_value=1  v_nominal_unit=V  T_specify=off  T_priority=None  T=300 K  T_nominal_specify=off  T_nominal_value=1  T_nominal_unit=K
  In : PMIOPort  Side=Left
  ~ : PMIOPort  Port=2  Side=Right
  wires:
  Data Type Conversion/1 -> Open Resistance/1
  BRK/1 -> Data Type Conversion/1
  Open Resistance/1 -> Simulink-PS Converter/1
  connections:
  Phase Splitter1/RConn2 -- Variable Resistor1/RConn1
  Variable Resistor1/LConn2 -- Phase Splitter/RConn2
  Phase Splitter1/RConn3 -- Variable Resistor2/RConn1
  Phase Splitter/RConn1 -- Variable Resistor/LConn2
  Variable Resistor2/LConn2 -- Phase Splitter/RConn3
  Phase Splitter1/RConn1 -- Variable Resistor/RConn1
  Phase Splitter1/LConn1 -- ~/RConn1
  Variable Resistor/LConn1 -- Simulink-PS Converter/RConn1 -- Variable Resistor2/LConn1 -- Variable Resistor1/LConn1
  Phase Splitter/LConn1 -- In/RConn1

== system IndustrialMicrogrid/MG2 PV Plant/PLL & Measurements2 ==
  V : Inport
  Measurement2 : Subsystem
  PLL : Subsystem
  Out Bus Element : Outport  PortName=Vbus  Element=Vq
  Out Bus Element1 : Outport  PortName=Vbus  Element=Vd
  Out Bus Element2 : Outport  PortName=Vbus  Element=w
  Out Bus Element3 : Outport  PortName=Vbus  Element=Theta
  Out Bus Element4 : Outport  PortName=Vbus  Element=Vmag
  wires:
  V/1 -> Measurement2/1(u)
  PLL/2(freq) -> Out Bus Element2/1
  PLL/5(Vq) -> Out Bus Element/1
  PLL/3(angle) -> Out Bus Element3/1
  PLL/4(Vd) -> Out Bus Element1/1
  Measurement2/1(Vg) -> PLL/1(abc)
  PLL/1(mag) -> Out Bus Element4/1

== system IndustrialMicrogrid/MG2 Power Center/Circuit Breaker ==
  BRK : Inport
  Data Type Conversion : DataTypeConversion  OutDataTypeStr=double  SaturateOnIntegerOverflow=off  RndMeth=Floor
  Open Resistance : Gain  Gain=1e5
  Phase Splitter : ee_lib/Connectors & References/Phase Splitter
  Phase Splitter1 : ee_lib/Connectors & References/Phase Splitter
  Simulink-PS Converter : nesl_utility/Simulink-PS Converter  PhysicalDomain=network_engine_domain  SubClassName=ps_input  LeftPortType=input  RightPortType=output  PseudoPeriodic=off  Frequencies=[]  NoiseDistribution=none  NoiseParameters=[]  Unit=1  AffineConversion=off  FilteringAndDerivatives=provide  SimscapeFilterOrder=1  InputFilterTimeConstant=0.001  UdotUserProvided=0
  Variable Resistor : fl_lib/Electrical/Electrical Elements/Variable Resistor  Rmin=1e-3 Ohm  thermalEnable=false  thermal_mass=1 J/K  i_specify=off  i_priority=None  i=0 A  i_nominal_specify=off  i_nominal_value=1  i_nominal_unit=A  v_specify=off  v_priority=None  v=0 V  v_nominal_specify=off  v_nominal_value=1  v_nominal_unit=V  T_specify=off  T_priority=None  T=300 K  T_nominal_specify=off  T_nominal_value=1  T_nominal_unit=K
  Variable Resistor1 : fl_lib/Electrical/Electrical Elements/Variable Resistor  Rmin=1e-3 Ohm  thermalEnable=false  thermal_mass=1 J/K  i_specify=off  i_priority=None  i=0 A  i_nominal_specify=off  i_nominal_value=1  i_nominal_unit=A  v_specify=off  v_priority=None  v=0 V  v_nominal_specify=off  v_nominal_value=1  v_nominal_unit=V  T_specify=off  T_priority=None  T=300 K  T_nominal_specify=off  T_nominal_value=1  T_nominal_unit=K
  Variable Resistor2 : fl_lib/Electrical/Electrical Elements/Variable Resistor  Rmin=1e-3 Ohm  thermalEnable=false  thermal_mass=1 J/K  i_specify=off  i_priority=None  i=0 A  i_nominal_specify=off  i_nominal_value=1  i_nominal_unit=A  v_specify=off  v_priority=None  v=0 V  v_nominal_specify=off  v_nominal_value=1  v_nominal_unit=V  T_specify=off  T_priority=None  T=300 K  T_nominal_specify=off  T_nominal_value=1  T_nominal_unit=K
  In : PMIOPort  Side=Left
  ~ : PMIOPort  Port=2  Side=Right
  wires:
  Data Type Conversion/1 -> Open Resistance/1
  BRK/1 -> Data Type Conversion/1
  Open Resistance/1 -> Simulink-PS Converter/1
  connections:
  Phase Splitter1/RConn2 -- Variable Resistor1/RConn1
  Variable Resistor1/LConn2 -- Phase Splitter/RConn2
  Phase Splitter1/RConn3 -- Variable Resistor2/RConn1
  Phase Splitter/RConn1 -- Variable Resistor/LConn2
  Variable Resistor2/LConn2 -- Phase Splitter/RConn3
  Phase Splitter1/RConn1 -- Variable Resistor/RConn1
  Phase Splitter1/LConn1 -- ~/RConn1
  Variable Resistor/LConn1 -- Simulink-PS Converter/RConn1 -- Variable Resistor2/LConn1 -- Variable Resistor1/LConn1
  Phase Splitter/LConn1 -- In/RConn1

== system IndustrialMicrogrid/MG2 Power Center/Circuit Breaker1 ==
  BRK : Inport
  Data Type Conversion : DataTypeConversion  OutDataTypeStr=double  SaturateOnIntegerOverflow=off  RndMeth=Floor
  Open Resistance : Gain  Gain=1e5
  Phase Splitter : ee_lib/Connectors & References/Phase Splitter
  Phase Splitter1 : ee_lib/Connectors & References/Phase Splitter
  Simulink-PS Converter : nesl_utility/Simulink-PS Converter  PhysicalDomain=network_engine_domain  SubClassName=ps_input  LeftPortType=input  RightPortType=output  PseudoPeriodic=off  Frequencies=[]  NoiseDistribution=none  NoiseParameters=[]  Unit=1  AffineConversion=off  FilteringAndDerivatives=provide  SimscapeFilterOrder=1  InputFilterTimeConstant=0.001  UdotUserProvided=0
  Variable Resistor : fl_lib/Electrical/Electrical Elements/Variable Resistor  Rmin=1e-3 Ohm  thermalEnable=false  thermal_mass=1 J/K  i_specify=off  i_priority=None  i=0 A  i_nominal_specify=off  i_nominal_value=1  i_nominal_unit=A  v_specify=off  v_priority=None  v=0 V  v_nominal_specify=off  v_nominal_value=1  v_nominal_unit=V  T_specify=off  T_priority=None  T=300 K  T_nominal_specify=off  T_nominal_value=1  T_nominal_unit=K
  Variable Resistor1 : fl_lib/Electrical/Electrical Elements/Variable Resistor  Rmin=1e-3 Ohm  thermalEnable=false  thermal_mass=1 J/K  i_specify=off  i_priority=None  i=0 A  i_nominal_specify=off  i_nominal_value=1  i_nominal_unit=A  v_specify=off  v_priority=None  v=0 V  v_nominal_specify=off  v_nominal_value=1  v_nominal_unit=V  T_specify=off  T_priority=None  T=300 K  T_nominal_specify=off  T_nominal_value=1  T_nominal_unit=K
  Variable Resistor2 : fl_lib/Electrical/Electrical Elements/Variable Resistor  Rmin=1e-3 Ohm  thermalEnable=false  thermal_mass=1 J/K  i_specify=off  i_priority=None  i=0 A  i_nominal_specify=off  i_nominal_value=1  i_nominal_unit=A  v_specify=off  v_priority=None  v=0 V  v_nominal_specify=off  v_nominal_value=1  v_nominal_unit=V  T_specify=off  T_priority=None  T=300 K  T_nominal_specify=off  T_nominal_value=1  T_nominal_unit=K
  In : PMIOPort  Side=Left
  ~ : PMIOPort  Port=2  Side=Right
  wires:
  Data Type Conversion/1 -> Open Resistance/1
  BRK/1 -> Data Type Conversion/1
  Open Resistance/1 -> Simulink-PS Converter/1
  connections:
  Phase Splitter1/RConn2 -- Variable Resistor1/RConn1
  Variable Resistor1/LConn2 -- Phase Splitter/RConn2
  Phase Splitter1/RConn3 -- Variable Resistor2/RConn1
  Phase Splitter/RConn1 -- Variable Resistor/LConn2
  Variable Resistor2/LConn2 -- Phase Splitter/RConn3
  Phase Splitter1/RConn1 -- Variable Resistor/RConn1
  Phase Splitter1/LConn1 -- ~/RConn1
  Variable Resistor/LConn1 -- Simulink-PS Converter/RConn1 -- Variable Resistor2/LConn1 -- Variable Resistor1/LConn1
  Phase Splitter/LConn1 -- In/RConn1

== system IndustrialMicrogrid/MG2 Power Center/Circuit Breaker3 ==
  BRK : Inport
  Data Type Conversion : DataTypeConversion  OutDataTypeStr=double  SaturateOnIntegerOverflow=off  RndMeth=Floor
  Open Resistance : Gain  Gain=1e6
  Phase Splitter : ee_lib/Connectors & References/Phase Splitter
  Phase Splitter1 : ee_lib/Connectors & References/Phase Splitter
  Simulink-PS Converter : nesl_utility/Simulink-PS Converter  PhysicalDomain=network_engine_domain  SubClassName=ps_input  LeftPortType=input  RightPortType=output  PseudoPeriodic=off  Frequencies=[]  NoiseDistribution=none  NoiseParameters=[]  Unit=1  AffineConversion=off  FilteringAndDerivatives=provide  SimscapeFilterOrder=1  InputFilterTimeConstant=0.001  UdotUserProvided=0
  Variable Resistor : fl_lib/Electrical/Electrical Elements/Variable Resistor  Rmin=1e-3 Ohm  thermalEnable=false  thermal_mass=1 J/K  i_specify=off  i_priority=None  i=0 A  i_nominal_specify=off  i_nominal_value=1  i_nominal_unit=A  v_specify=off  v_priority=None  v=0 V  v_nominal_specify=off  v_nominal_value=1  v_nominal_unit=V  T_specify=off  T_priority=None  T=300 K  T_nominal_specify=off  T_nominal_value=1  T_nominal_unit=K
  Variable Resistor1 : fl_lib/Electrical/Electrical Elements/Variable Resistor  Rmin=1e-3 Ohm  thermalEnable=false  thermal_mass=1 J/K  i_specify=off  i_priority=None  i=0 A  i_nominal_specify=off  i_nominal_value=1  i_nominal_unit=A  v_specify=off  v_priority=None  v=0 V  v_nominal_specify=off  v_nominal_value=1  v_nominal_unit=V  T_specify=off  T_priority=None  T=300 K  T_nominal_specify=off  T_nominal_value=1  T_nominal_unit=K
  Variable Resistor2 : fl_lib/Electrical/Electrical Elements/Variable Resistor  Rmin=1e-3 Ohm  thermalEnable=false  thermal_mass=1 J/K  i_specify=off  i_priority=None  i=0 A  i_nominal_specify=off  i_nominal_value=1  i_nominal_unit=A  v_specify=off  v_priority=None  v=0 V  v_nominal_specify=off  v_nominal_value=1  v_nominal_unit=V  T_specify=off  T_priority=None  T=300 K  T_nominal_specify=off  T_nominal_value=1  T_nominal_unit=K
  In : PMIOPort  Side=Left
  ~ : PMIOPort  Port=2  Side=Right
  wires:
  Data Type Conversion/1 -> Open Resistance/1
  BRK/1 -> Data Type Conversion/1
  Open Resistance/1 -> Simulink-PS Converter/1
  connections:
  Phase Splitter1/RConn2 -- Variable Resistor1/RConn1
  Variable Resistor1/LConn2 -- Phase Splitter/RConn2
  Phase Splitter1/RConn3 -- Variable Resistor2/RConn1
  Phase Splitter/RConn1 -- Variable Resistor/LConn2
  Variable Resistor2/LConn2 -- Phase Splitter/RConn3
  Phase Splitter1/RConn1 -- Variable Resistor/RConn1
  Phase Splitter1/LConn1 -- ~/RConn1
  Variable Resistor/LConn1 -- Simulink-PS Converter/RConn1 -- Variable Resistor2/LConn1 -- Variable Resistor1/LConn1
  Phase Splitter/LConn1 -- In/RConn1
